simulink subsystem "Block_DC"  (R2022a)
settings: Solver=VariableStepAuto  StartTime=0.0  StopTime=10.0  RelTol=1e-3
settings Model: Creator=mmarq  LastModifiedBy=mmarq

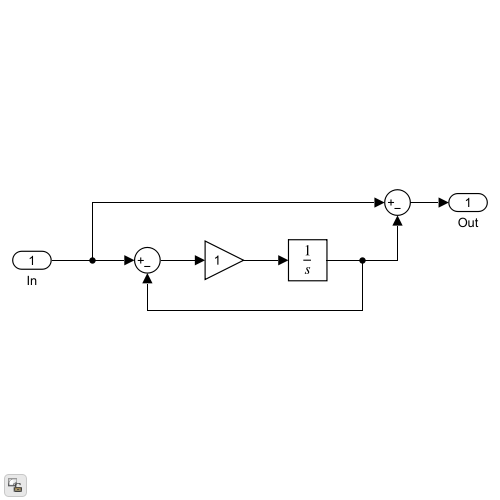
[thumbnail: Simulink's stored preview of the top-level diagram]
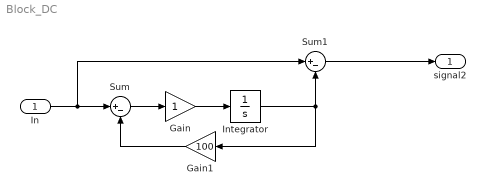
== system Block_DC ==
  In : Inport
  Gain : Gain
  Gain1 : Gain  Gain=100
  Integrator : Integrator
  Sum : Sum  Inputs=|+-
  Sum1 : Sum  Inputs=|+-
  signal2 : Outport
  wires:
  Gain/1 -> Integrator/1
  Sum/1 -> Gain/1
  Integrator/1 -> Gain1/1, Sum1/2
  Sum1/1 -> signal2/1
  In/1 -> Sum/1, Sum1/1
  Gain1/1 -> Sum/2
